simulink model "KR6_dynamics"  (R2018a)
settings: Solver=VariableStepAuto  StartTime=0.0  StopTime=inf  RelTol=1e-3
libraries: vrlib x8, dspinverses x1, realtime_pacer_lib x1
(part 1 of 2)
settings Model: Creator=Pedro Ramalho  LastModifiedBy=Pedro Ramalho

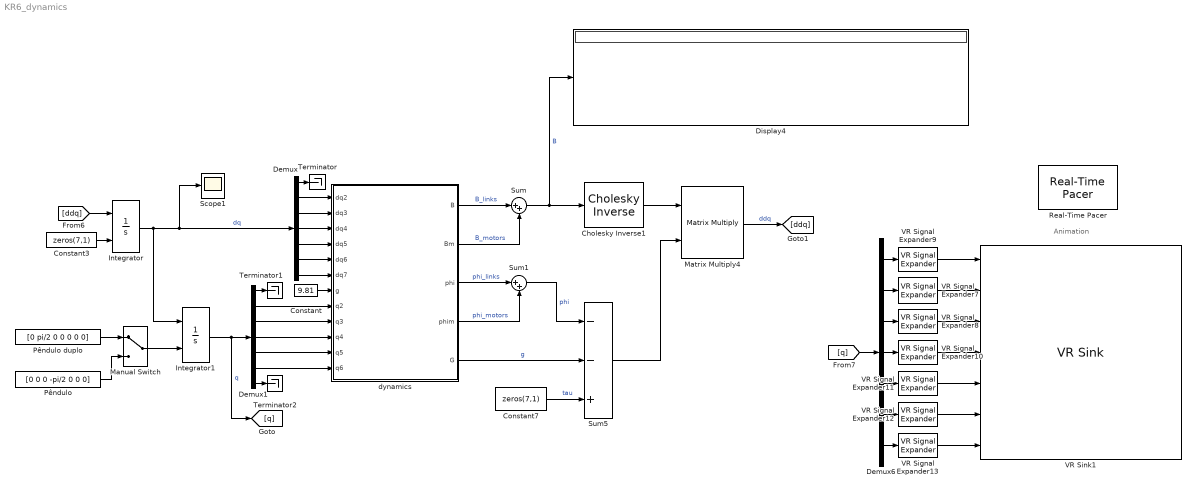
== system KR6_dynamics ==
  note: Animation
  Cholesky Inverse1 : dspinverses/Cholesky Inverse  errmode=Warning
      settings: SourceProductName=DSP System Toolbox  SourceProductBaseCode=DS
  Constant : Constant  Value=9.81  SampleTime=-1
  Constant3 : Constant  Value=zeros(7,1)  SampleTime=-1
  Constant7 : Constant  Value=zeros(7,1)  SampleTime=-1
  Demux : Demux  Outputs=7
  Demux1 : Demux  Outputs=7
  Demux6 : Demux  Outputs=7
  Display4 : Display
  Integrator : Integrator  InitialConditionSource=external
  Integrator1 : Integrator  InitialConditionSource=external
  Manual Switch : ManualSwitch
  Matrix Multiply4 : Product  Multiplication=Matrix(*)
  Pêndulo : Constant  Value=[0 0 0 -pi/2 0 0 0]  SampleTime=-1
  Pêndulo duplo : Constant  Value=[0 pi/2 0 0 0 0 0]  SampleTime=-1
  Real-Time Pacer : realtime_pacer_lib/Real-Time Pacer  simTimePerRealTime=1
  Scope1 : Scope
  Sum : Sum  Inputs=|++
  Sum1 : Sum  Inputs=|++
  Sum5 : Sum  Inputs=--+
  Terminator : Terminator
  Terminator1 : Terminator
  Terminator2 : Terminator
  VR Signal Expander{7..8,10..13} (6 alike) : vrlib/VR Signal Expander  outwidth=4  outidx=4
      settings: SourceProductName=Simulink 3D Animation  SourceProductBaseCode=VR
  VR Signal Expander9 : vrlib/VR Signal Expander  outwidth=3  outidx=3
      settings: SourceProductName=Simulink 3D Animation  SourceProductBaseCode=VR
  VR Sink1 : vrlib/VR Sink  InstantiateOnLoad=on  SampleTime=0.1  ViewEnable=on  RemoteChange=off  RemoteView=off  FieldsWritten=Jt1_DH_dv.translation.3.1.1.double#Jt2_DH_dv.rotation.4.1.1.double#Jt3_DH_dv.rotation.4.1.1.double#Jt4_DH_dv.rotation.4.1.1.double#Jt5_DH_dv.rotation.4.1.1.double#Jt6_DH_dv.rotation.4.1.1.double#Jt7_DH_dv.rotation.4.1.1.double  WorldFileName=vrrobotKR6.wrl  WorldDescription=D-H Reference Frames for Virtual Reality Robot  AutoView=off  VideoDimensions=[]  AllowVariableSize=off  FigureProperties="{'Position', 'Name', 'Viewpoint', 'CameraBound', 'CameraDirection', 'CameraPosition', 'CameraUpVector', 'ZoomFactor', 'Antialiasing', 'Headlight', 'Lighting', 'NavPanel', 'Sound', 'StatusBar', 'Stereo3D', 'Stereo3DCameraOffset', 'Stereo3DHIT', 'ToolBar', 'Textures', 'Transparency', 'Triad', 'Wireframe', 'NavZones', 'NavMode', 'NavSpeed', 'CaptureFileFormat', 'CaptureFileName', 'Record2DCompressMethod', 'Record2DCompressQuality', 'Record2D', 'Record2DFileName', 'Record2DFPS'; [5.0000000000000000e+00   9.2000000000000000e+01   5.7600000000000000e+02   3.5000000000000000e+02], 'D-H Reference Frames for Virtual Reality Robot', 'View 1', 'on', [0.0000000000000000e+00   9.0044696580978023e-01  -4.3496581677638979e-01], [0.0000000000000000e+00  -4.1000065564843569e+00  -1.8999841924381577e+00], [0.0000000000000000e+00   4.3496581677638979e-01   9.0044696580978023e-01], [1.0000000000000000e+00], 'on', 'on', 'on', 'halfbar', 'on', 'on', 'off', [1.0000000149011612e-01], [0.0000000000000000e+00], 'on', 'on', 'on', 'none', 'off', 'off', 'examine', 'normal', 'tif', '%f_anim_%n.tif', 'auto', [7.5000000000000000e+01], 'off', '%f_anim_%n.avi', 'auto'}"
      settings: SourceProductBaseCode=VR
  dynamics : MATLAB Function  TreatAsAtomicUnit=on
  wires:
  dynamics/1(B) -> Sum/1  "B_links"
  dynamics/2(Bm) -> Sum/2  "B_motors"
  Sum/1 -> Cholesky Inverse1/1, Display4/1  "B"
  Sum1/1 -> Sum5/1  "phi"
  dynamics/3(phi) -> Sum1/1  "phi_links"
  dynamics/4(phim) -> Sum1/2  "phi_motors"
  dynamics/5(G) -> Sum5/2  "g"
  Demux/2 -> dynamics/1(dq2)
  Demux/3 -> dynamics/2(dq3)
  Demux/4 -> dynamics/3(dq4)
  Demux/5 -> dynamics/4(dq5)
  Demux/6 -> dynamics/5(dq6)
  Demux/7 -> dynamics/6(dq7)
  Demux/1 -> Terminator/1
  Demux1/7 -> Terminator2/1
  Demux1/6 -> dynamics/12(q6)
  Demux1/5 -> dynamics/11(q5)
  Demux1/1 -> Terminator1/1
  Demux1/2 -> dynamics/8(q2)
  Demux1/4 -> dynamics/10(q4)
  Demux1/3 -> dynamics/9(q3)
  Constant/1 -> dynamics/7(g)
  Integrator1/1 -> Demux1/1, [q]  "q"
  Integrator/1 -> Integrator1/1, Scope1/1, Demux/1  "dq"
  Constant3/1 -> Integrator/2
  Constant7/1 -> Sum5/3  "tau"
  Cholesky Inverse1/1 -> Matrix Multiply4/1
  Sum5/1 -> Matrix Multiply4/2
  VR Signal Expander11/1 -> VR Sink1/5
  [q] -> Demux6/1
  Demux6/3 -> VR Signal Expander8/1
  Demux6/2 -> VR Signal Expander7/1
  Demux6/7 -> VR Signal Expander13/1
  VR Signal Expander10/1 -> VR Sink1/4
  Demux6/1 -> VR Signal Expander9/1
  VR Signal Expander8/1 -> VR Sink1/3
  VR Signal Expander7/1 -> VR Sink1/2
  Demux6/4 -> VR Signal Expander10/1
  Demux6/5 -> VR Signal Expander11/1
  Demux6/6 -> VR Signal Expander12/1
  VR Signal Expander13/1 -> VR Sink1/7
  VR Signal Expander12/1 -> VR Sink1/6
  VR Signal Expander9/1 -> VR Sink1/1
  Matrix Multiply4/1 -> [ddq]  "ddq"
  [ddq] -> Integrator/1
  Manual Switch/1 -> Integrator1/2
  Pêndulo duplo/1 -> Manual Switch/1
  Pêndulo/1 -> Manual Switch/2
